simulink model "heading_nomoto1_controller"  (R2017b)
settings: Solver=VariableStepAuto  StartTime=0.0  StopTime=tstop  RelTol=1e-3
values from neighbouring files (symbols this model uses):
  K1 = 0.00466/dc    (= 0.088999444177)    [TTK4190_A3_task1_2.m]    (also in TTK4190_A3_task1_3.m = 0.089; parameters_heading_controller.m = 0.089)
  Kd_psi = 150    [TTK4190_A3_task1_3.m]    (also in parameters_heading_controller.m)
  Ki_psi = 0.025/10*Kp_psi/5    (= 0.0004)    [TTK4190_A3_task1_3.m]    (also in parameters_heading_controller.m)
  Kp_psi = 0.8    [TTK4190_A3_task1_3.m]    (also in parameters_heading_controller.m)
  psi_d = 5*deg2rad    (= 0.0872664625997)    [TTK4190_A3_task1_2.m]    (also in TTK4190_A3_task1_3.m = 0.13962634016; model_analysis.m = 0.13962634016; parameters_heading_controller.m = 0.13962634016)
  r_d = 0*deg2rad    (= 0)    [TTK4190_A3_task1_3.m]    (also in parameters_heading_controller.m)
  T = 197.5    [TTK4190_A3_task1_2.m]    (also in TTK4190_A3_task1_3.m; model_analysis.m = x(1); parameters_heading_controller.m)
  tsamp = 10    [TTK4190_A3_task1_2.m]    (also in TTK4190_A3_task1_3.m; model_analysis.m = 35; sim_nomoto2.m = tsamp; sysID.m = 100)
undefined symbols (not defined in the file or in its folder): Ki_r, Kp_r
settings Model: Creator=Marie  LastModifiedBy=Marie

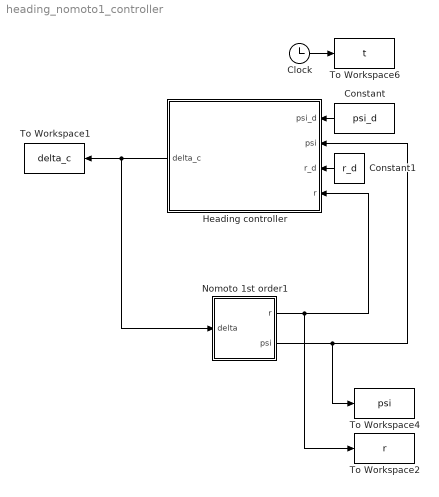
== system heading_nomoto1_controller ==
  Clock : Clock
  Constant : Constant  Value=psi_d
  Constant1 : Constant  Value=r_d
  Heading controller : Subsystem
  Nomoto 1st order1 : Subsystem
  To Workspace1 : ToWorkspace  VariableName=delta_c  SampleTime=tsamp
  To Workspace2 : ToWorkspace  VariableName=r  SampleTime=tsamp
  To Workspace4 : ToWorkspace  VariableName=psi  SampleTime=tsamp
  To Workspace6 : ToWorkspace  VariableName=t  SampleTime=tsamp
  wires:
  Heading controller/1(delta_c) -> To Workspace1/1, Nomoto 1st order1/1(delta)
  Nomoto 1st order1/1(r) -> To Workspace2/1, Heading controller/4(r)
  Nomoto 1st order1/2(psi) -> To Workspace4/1, Heading controller/2(psi)
  Constant/1 -> Heading controller/1("psi_d ")
  Constant1/1 -> Heading controller/3(r_d)
  Clock/1 -> To Workspace6/1

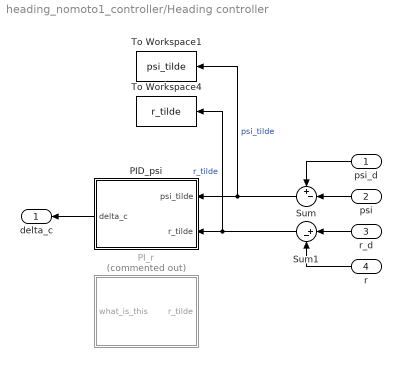
== system heading_nomoto1_controller/Heading controller ==
  "psi_d " : Inport
  psi : Inport  Port=2
  r_d : Inport  Port=3
  r : Inport  Port=4
  PID_psi : Subsystem
  PI_r : Subsystem  Commented=on
  Sum : Sum  Inputs=+-|
  Sum1 : Sum  Inputs=|+-
  To Workspace1 : ToWorkspace  VariableName=psi_tilde  SampleTime=tsamp
  To Workspace4 : ToWorkspace  VariableName=r_tilde  SampleTime=tsamp
  delta_c : Outport
  wires:
  PID_psi/1(delta_c) -> delta_c/1
  psi/1 -> Sum/2
  "psi_d "/1 -> Sum/1
  Sum1/1 -> To Workspace4/1, PID_psi/2(r_tilde)  "r_tilde"
  r_d/1 -> Sum1/1
  r/1 -> Sum1/2
  Sum/1 -> To Workspace1/1, PID_psi/1(psi_tilde)  "psi_tilde"

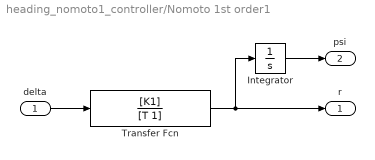
== system heading_nomoto1_controller/Nomoto 1st order1 ==
  delta : Inport
  Integrator : Integrator
  Transfer Fcn : TransferFcn  Numerator=[K1]  Denominator=[T 1]
  r : Outport
  psi : Outport  Port=2
  wires:
  delta/1 -> Transfer Fcn/1
  Transfer Fcn/1 -> Integrator/1, r/1
  Integrator/1 -> psi/1

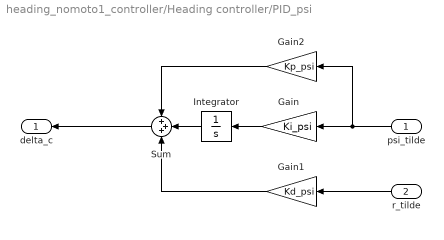
== system heading_nomoto1_controller/Heading controller/PID_psi ==
  psi_tilde : Inport
  r_tilde : Inport  Port=2
  Gain : Gain  Gain=Ki_psi
  Gain1 : Gain  Gain=Kd_psi
  Gain2 : Gain  Gain=Kp_psi
  Integrator : Integrator
  Sum : Sum  Inputs=+++
  delta_c : Outport
  wires:
  Gain2/1 -> Sum/1
  r_tilde/1 -> Gain1/1
  Gain1/1 -> Sum/3
  psi_tilde/1 -> Gain2/1, Gain/1
  Sum/1 -> delta_c/1
  Gain/1 -> Integrator/1
  Integrator/1 -> Sum/2

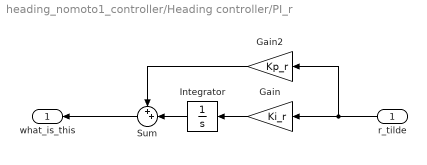
== system heading_nomoto1_controller/Heading controller/PI_r ==
  r_tilde : Inport
  Gain : Gain  Gain=Ki_r
  Gain2 : Gain  Gain=Kp_r
  Integrator : Integrator
  Sum : Sum  Inputs=++|
  what_is_this : Outport
  wires:
  Gain2/1 -> Sum/1
  r_tilde/1 -> Gain2/1, Gain/1
  Sum/1 -> what_is_this/1
  Gain/1 -> Integrator/1
  Integrator/1 -> Sum/2
